simulink model "Frenet_Coordinate_State"  (R2021b)
settings: Solver=VariableStepAuto  StartTime=0.0  StopTime=10.0  RelTol=1e-3
libraries: PreScanUsefulBlocks x1, simulink x1
settings Model: Creator=admin  LastModifiedBy=admin

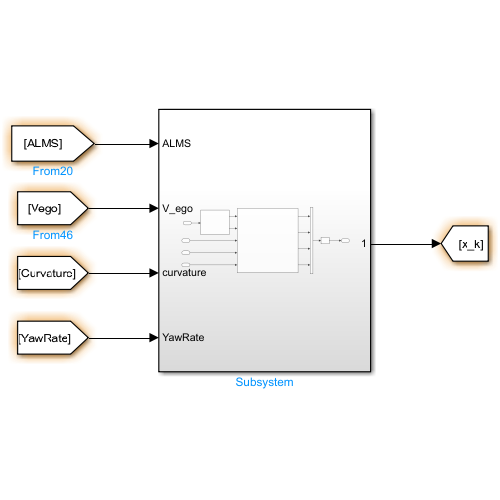
[thumbnail: Simulink's stored preview of the top-level diagram]
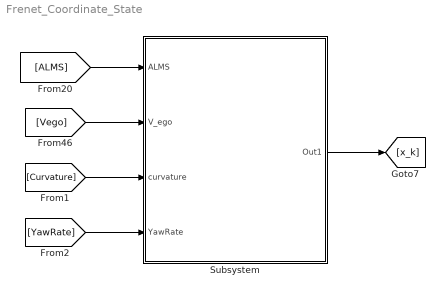
== system Frenet_Coordinate_State ==
  Subsystem : Subsystem
  wires:
  [ALMS] -> Subsystem/1(ALMS)
  [Vego] -> Subsystem/2(V_ego)
  [Curvature] -> Subsystem/3(curvature)
  [YawRate] -> Subsystem/4(YawRate)
  Subsystem/1(Out1) -> [x_k]

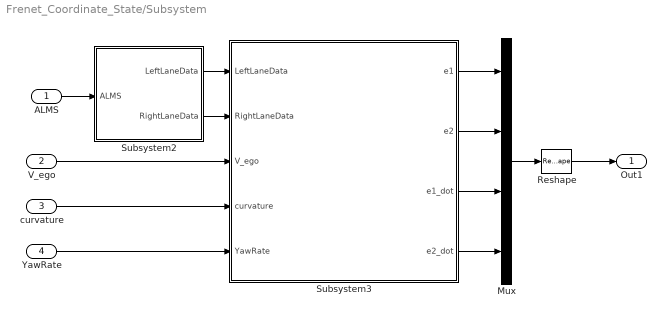
== system Frenet_Coordinate_State/Subsystem ==
  ALMS : Inport
  V_ego : Inport  Port=2
  curvature : Inport  Port=3
  YawRate : Inport  Port=4
  Mux : Mux
  Reshape : Reshape  OutputDimensionality=Customize  OutputDimensions=[4,1]
  Subsystem2 : Subsystem
  Subsystem3 : Subsystem
  Out1 : Outport
  wires:
  Subsystem3/1(e1) -> Mux/1
  Reshape/1 -> Out1/1
  Subsystem3/3(e1_dot) -> Mux/3
  Subsystem3/4(e2_dot) -> Mux/4
  Subsystem2/2(RightLaneData) -> Subsystem3/2(RightLaneData)
  Subsystem3/2(e2) -> Mux/2
  Mux/1 -> Reshape/1
  Subsystem2/1(LeftLaneData) -> Subsystem3/1(LeftLaneData)
  YawRate/1 -> Subsystem3/5(YawRate)
  V_ego/1 -> Subsystem3/3(V_ego)
  ALMS/1 -> Subsystem2/1(ALMS)
  curvature/1 -> Subsystem3/4(curvature)

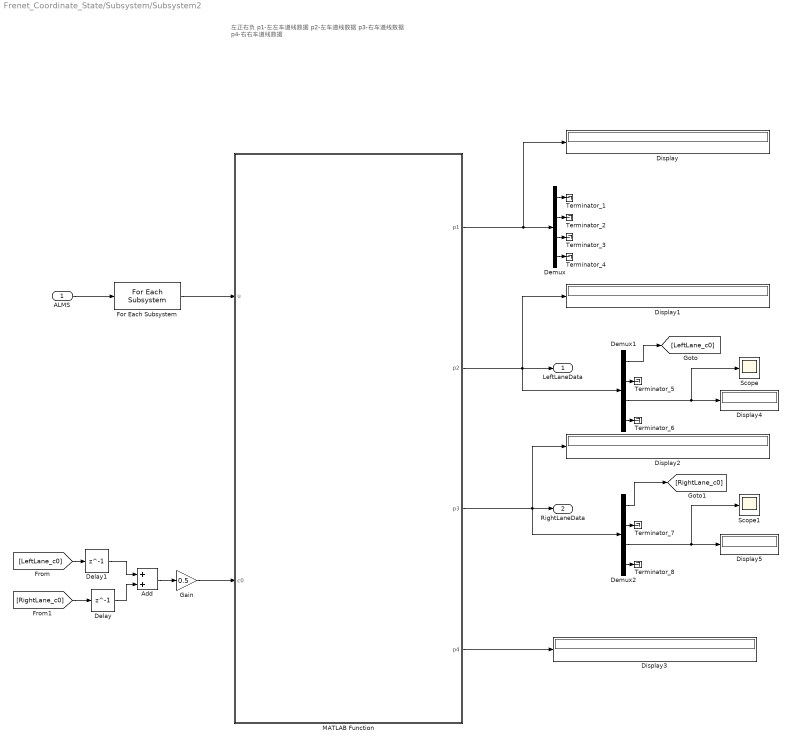
== system Frenet_Coordinate_State/Subsystem/Subsystem2 ==
  note: 左正右负
      | p1-左左车道线数据
      | p2-左车道线数据
      | p3-右车道线数据
      | p4-右右车道线数据
  ALMS : Inport  OutDataTypeStr=Bus: PRESCAN_ALMS_MESSAGE
  Add : Sum
  Delay : Delay  DelayLength=1
  Delay1 : Delay  DelayLength=1
  Demux : Demux
  Demux1 : Demux
  Demux2 : Demux
  Display{,1..5} (6 alike) : Display
  For Each Subsystem : PreScanUsefulBlocks/ALMS XY Polynomial Plot/For Each Subsystem  SystemSampleTime=-1  VariantActivationTime=update diagram  Latency=0  AutoFrameSizeCalculation=off
  Gain : Gain  Gain=0.5
  MATLAB Function : MATLAB Function  TreatAsAtomicUnit=on
  Scope : Scope
  Scope1 : Scope
  Terminator_{1..8} (8 alike) : Terminator
  LeftLaneData : Outport  VectorParamsAs1DForOutWhenUnconnected=off
  RightLaneData : Outport  Port=2  VectorParamsAs1DForOutWhenUnconnected=off
  wires:
  For Each Subsystem/1 -> MATLAB Function/1(u)
  ALMS/1 -> For Each Subsystem/1
  Gain/1 -> MATLAB Function/2(c0)
  Demux1/3 -> Scope/1, Display4/1
  Demux2/3 -> Scope1/1, Display5/1
  Demux1/1 -> [LeftLane_c0]
  Demux2/1 -> [RightLane_c0]
  [LeftLane_c0] -> Delay1/1
  [RightLane_c0] -> Delay/1
  Add/1 -> Gain/1
  Delay1/1 -> Add/1
  Delay/1 -> Add/2
  MATLAB Function/2(p2) -> Demux1/1, LeftLaneData/1, Display1/1
  MATLAB Function/1(p1) -> Display/1, Demux/1
  MATLAB Function/3(p3) -> Demux2/1, RightLaneData/1, Display2/1
  MATLAB Function/4(p4) -> Display3/1
  Demux/1 -> Terminator_1/1
  Demux/2 -> Terminator_2/1
  Demux/3 -> Terminator_3/1
  Demux/4 -> Terminator_4/1
  Demux1/2 -> Terminator_5/1
  Demux1/4 -> Terminator_6/1
  Demux2/2 -> Terminator_7/1
  Demux2/4 -> Terminator_8/1

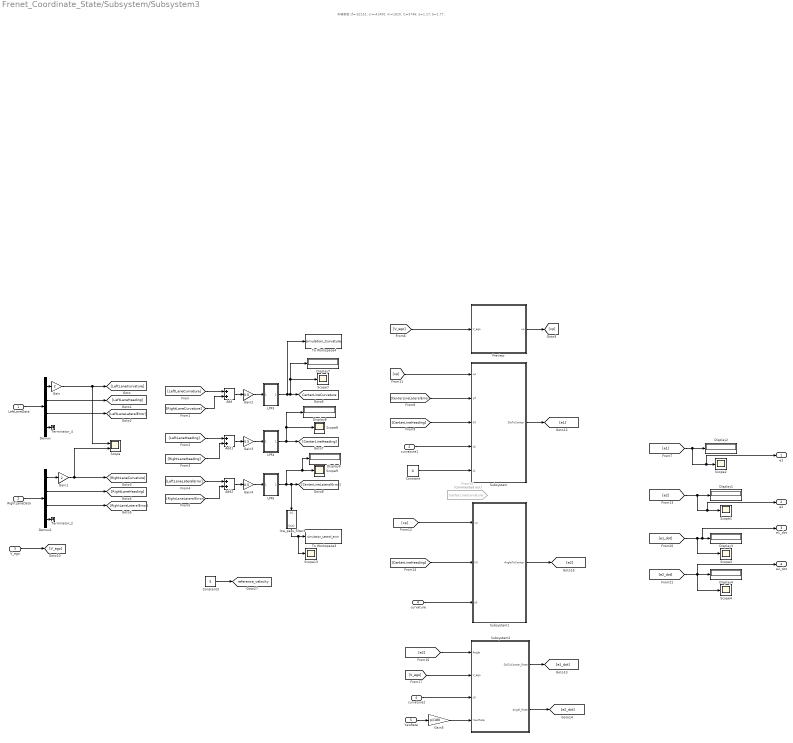
== system Frenet_Coordinate_State/Subsystem/Subsystem3 ==
  note: 车辆参数
      | cf=-52151;
      | cr=-41400;
      | m=1820;
      | Iz=3746;
      | a=1.17;
      | b=1.77;
  LeftLaneData : Inport
  RightLaneData : Inport  Port=2
  V_ego : Inport  Port=3
  curvature : Inport  Port=4
  YawRate : Inport  Port=5
  Add : Sum
  Add1 : Sum
  Add2 : Sum
  Constant : Constant  Value=0
  Constant3 : Constant  Value=5
  Demux : Demux
  Demux1 : Demux
  Display{1..4,7..9} (7 alike) : Display
  From10 : From  Commented=on  GotoTag=CenterLineCurvature  TagVisibility=global
  Gain : Gain  Gain=2
  Gain1 : Gain  Gain=2
  Gain2 : Gain  Gain=0.5
  Gain3 : Gain  Gain=0.5
  Gain4 : Gain  Gain=0.5
  Gain5 : Gain  Gain=pi/180
  LPF3 : Subsystem
  LPF4 : Subsystem
  LPF5 : Subsystem
  Preview : Subsystem
  Scope : Scope  NumInputPorts=2
  Scope{1..4,7..9,13} (8 alike) : Scope
  Subsystem : Subsystem
  Subsystem1 : Subsystem
  Subsystem2 : Subsystem
  Terminator_2 : Terminator
  Terminator_4 : Terminator
  To Workspace3 : ToWorkspace  VariableName=simulation_Lateral_error  SampleTime=-1
      settings: Save2DSignal=2-D array (concatenate along first dimension)
  To Workspace4 : ToWorkspace  VariableName=simulation_Curvature  SampleTime=-1
      settings: Save2DSignal=2-D array (concatenate along first dimension)
  curvature1 : InportShadow  Port=4
  curvature2 : InportShadow  Port=4
  low_pass_filter3 : Subsystem
  e1 : Outport
  e2 : Outport  Port=2
  e1_dot : Outport  Port=3
  e2_dot : Outport  Port=4
  tag scope: CenterLineCurvature=global, reference_velocity=global
  wires:
  LeftLaneData/1 -> Demux/1
  RightLaneData/1 -> Demux1/1
  Demux/1 -> Gain/1
  Demux1/1 -> Gain1/1
  [LeftLaneCurvature] -> Add/1
  [RightLaneCurvature] -> Add/2
  Add/1 -> Gain2/1
  Gain2/1 -> LPF3/1(In1)
  Add1/1 -> Gain3/1
  [LeftLaneHeading] -> Add1/1
  [RightLaneHeading] -> Add1/2
  [LeftLaneLateralError] -> Add2/1
  [RightLaneLateralError] -> Add2/2
  Add2/1 -> Gain4/1
  V_ego/1 -> [V_ego]
  [V_ego] -> Preview/1(V_ego)
  [CenterLineLateralError] -> Subsystem/2(y0)
  [CenterLineHeading] -> Subsystem/3(k0)
  Constant/1 -> Subsystem/5(c1)
  [xp] -> Subsystem/1(xp)
  [xp] -> Subsystem1/1(xp)
  [CenterLineHeading] -> Subsystem1/2(k0)
  [e2] -> Subsystem2/1(Angle)
  [V_ego] -> Subsystem2/2("V_ego ")
  YawRate/1 -> Gain5/1
  Subsystem/1(DisToCenter) -> [e1]
  Subsystem1/1(AngleToCenter) -> [e2]
  Subsystem2/1(DisToCenter_Rate) -> [e1_dot]
  Subsystem2/2(Angel_Rate) -> [e2_dot]
  Gain3/1 -> LPF4/1(In1)
  Gain4/1 -> LPF5/1(In1)
  Gain/1 -> Scope/1, [LeftLaneCurvature]
  Demux/2 -> [LeftLaneHeading]
  Demux/3 -> [LeftLaneLateralError]
  Gain1/1 -> Scope/2, [RightLaneCurvature]
  Demux1/2 -> [RightLaneHeading]
  Demux1/3 -> [RightLaneLateralError]
  LPF3/1(Out1) -> To Workspace4/1, Display7/1, Scope7/1, [CenterLineCurvature]
  LPF4/1(Out1) -> [CenterLineHeading], Display8/1, Scope8/1
  LPF5/1(Out1) -> [CenterLineLateralError], low_pass_filter3/1(In1), Display9/1, Scope9/1
  Demux/4 -> Terminator_4/1
  Demux1/4 -> Terminator_2/1
  Preview/1(xp) -> [xp]
  Gain5/1 -> Subsystem2/4(YawRate)
  low_pass_filter3/1(Out1) -> Scope13/1, To Workspace3/1
  Constant3/1 -> [reference_velocity]
  [e1] -> e1/1, Scope2/1, Display2/1
  [e2] -> Display1/1, e2/1, Scope1/1
  [e1_dot] -> Scope3/1, e1_dot/1, Display3/1
  [e2_dot] -> e2_dot/1, Display4/1, Scope4/1
  curvature1/1 -> Subsystem/4(c0)
  curvature/1 -> Subsystem1/3(c0)
  curvature2/1 -> Subsystem2/3(c0)

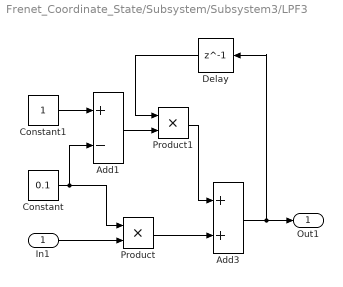
== system Frenet_Coordinate_State/Subsystem/Subsystem3/LPF3 ==
  In1 : Inport
  Add1 : Sum  Inputs=+-
  Add3 : Sum
  Constant : Constant  Value=0.1
  Constant1 : Constant
  Delay : Delay  DelayLength=1
  Product : Product
  Product1 : Product
  Out1 : Outport  VectorParamsAs1DForOutWhenUnconnected=off
  wires:
  In1/1 -> Product/2
  Add3/1 -> Delay/1, Out1/1
  Product/1 -> Add3/2
  Constant/1 -> Add1/2, Product/1
  Constant1/1 -> Add1/1
  Add1/1 -> Product1/2
  Delay/1 -> Product1/1
  Product1/1 -> Add3/1

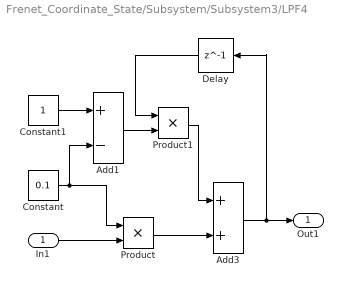
== system Frenet_Coordinate_State/Subsystem/Subsystem3/LPF4 ==
  In1 : Inport
  Add1 : Sum  Inputs=+-
  Add3 : Sum
  Constant : Constant  Value=0.1
  Constant1 : Constant
  Delay : Delay  DelayLength=1
  Product : Product
  Product1 : Product
  Out1 : Outport  VectorParamsAs1DForOutWhenUnconnected=off
  wires:
  Product1/1 -> Add3/1
  Delay/1 -> Product1/1
  Add1/1 -> Product1/2
  Constant1/1 -> Add1/1
  Constant/1 -> Product/1, Add1/2
  Product/1 -> Add3/2
  Add3/1 -> Out1/1, Delay/1
  In1/1 -> Product/2

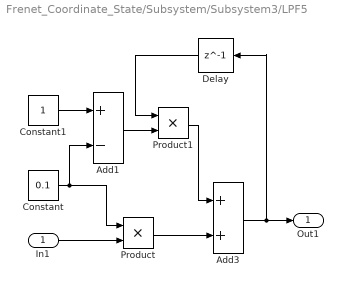
== system Frenet_Coordinate_State/Subsystem/Subsystem3/LPF5 ==
  In1 : Inport
  Add1 : Sum  Inputs=+-
  Add3 : Sum
  Constant : Constant  Value=0.1
  Constant1 : Constant
  Delay : Delay  DelayLength=1
  Product : Product
  Product1 : Product
  Out1 : Outport  VectorParamsAs1DForOutWhenUnconnected=off
  wires:
  In1/1 -> Product/2
  Add3/1 -> Delay/1, Out1/1
  Product/1 -> Add3/2
  Constant/1 -> Add1/2, Product/1
  Constant1/1 -> Add1/1
  Add1/1 -> Product1/2
  Delay/1 -> Product1/1
  Product1/1 -> Add3/1

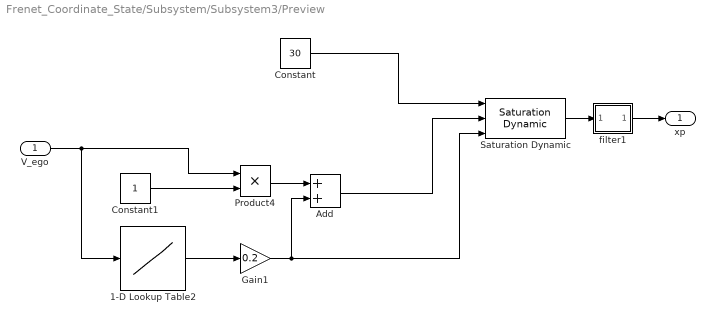
== system Frenet_Coordinate_State/Subsystem/Subsystem3/Preview ==
  V_ego : Inport
  1-D Lookup Table2 : Lookup_n-D  NumberOfTableDimensions=1  BreakpointsForDimension1=[0,3,5,10,15,20,30,40,50]  Table=[6,6,7,8.5,10.5,12,14,15,15]  InternalRulePriority=Speed  RndMeth=Simplest  InputSameDT=on
  Add : Sum
  Constant : Constant  Value=30
  Constant1 : Constant
  Gain1 : Gain  Gain=0.2
  Product4 : Product
  Saturation Dynamic : simulink/Discontinuities/Saturation Dynamic  OutMin=[]  OutMax=[]  OutDataTypeStr=Inherit: Same as second input  OutDataType=fixdt(1, 16)  OutScaling=2^-10  DoSatur=off
  filter1 : Subsystem
  xp : Outport  VectorParamsAs1DForOutWhenUnconnected=off
  wires:
  Constant/1 -> Saturation Dynamic/1
  Saturation Dynamic/1 -> filter1/1(In1)
  V_ego/1 -> 1-D Lookup Table2/1, Product4/1
  Product4/1 -> Add/1
  1-D Lookup Table2/1 -> Gain1/1
  Gain1/1 -> Add/2, Saturation Dynamic/3
  Constant1/1 -> Product4/2
  filter1/1(Out1) -> xp/1
  Add/1 -> Saturation Dynamic/2

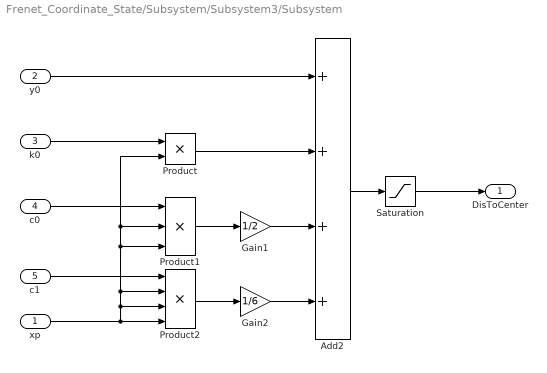
== system Frenet_Coordinate_State/Subsystem/Subsystem3/Subsystem ==
  xp : Inport
  y0 : Inport  Port=2
  k0 : Inport  Port=3
  c0 : Inport  Port=4
  c1 : Inport  Port=5
  Add2 : Sum  Inputs=++++
  Gain1 : Gain  Gain=1/2
  Gain2 : Gain  Gain=1/6
  Product : Product
  Product1 : Product  Inputs=3
  Product2 : Product  Inputs=4
  Saturation : Saturate  UpperLimit=3.5  LowerLimit=-3.5
  DisToCenter : Outport  VectorParamsAs1DForOutWhenUnconnected=off
  wires:
  Product1/1 -> Gain1/1
  Product2/1 -> Gain2/1
  Product/1 -> Add2/2
  c1/1 -> Product2/1
  Gain1/1 -> Add2/3
  Gain2/1 -> Add2/4
  c0/1 -> Product1/1
  Add2/1 -> Saturation/1
  xp/1 -> Product2/4, Product2/3, Product2/2, Product1/3, Product1/2, Product/2
  y0/1 -> Add2/1
  k0/1 -> Product/1
  Saturation/1 -> DisToCenter/1

== system Frenet_Coordinate_State/Subsystem/Subsystem3/Subsystem1 ==
  xp : Inport
  k0 : Inport  Port=2
  c0 : Inport  Port=3
  Add2 : Sum
  Product1 : Product
  Trigonometric Function : Trigonometry  Operator=atan
  AngleToCenter : Outport  VectorParamsAs1DForOutWhenUnconnected=off
  wires:
  Trigonometric Function/1 -> AngleToCenter/1
  c0/1 -> Product1/1
  Add2/1 -> Trigonometric Function/1
  Product1/1 -> Add2/2
  k0/1 -> Add2/1
  xp/1 -> Product1/2

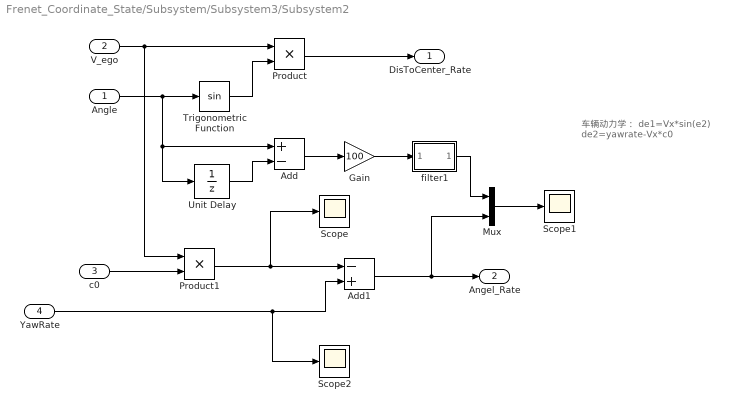
== system Frenet_Coordinate_State/Subsystem/Subsystem3/Subsystem2 ==
  note: 车辆动力学：
      | de1=Vx*sin(e2)
      | de2=yawrate-Vx*c0
  Angle : Inport
  "V_ego " : Inport  Port=2
  c0 : Inport  Port=3
  YawRate : Inport  Port=4
  Add : Sum  Inputs=+-
  Add1 : Sum  Inputs=-+
  Gain : Gain  Gain=100
  Mux : Mux  Inputs=2
  Product : Product
  Product1 : Product
  Scope : Scope
  Scope1 : Scope
  Scope2 : Scope
  Trigonometric Function : Trigonometry
  Unit Delay : UnitDelay  SampleTime=-1  HasFrameUpgradeWarning=on
  filter1 : Subsystem
  DisToCenter_Rate : Outport  VectorParamsAs1DForOutWhenUnconnected=off
  Angel_Rate : Outport  Port=2  VectorParamsAs1DForOutWhenUnconnected=off
  wires:
  "V_ego "/1 -> Product1/1, Product/1
  Angle/1 -> Unit Delay/1, Add/1, Trigonometric Function/1
  Product/1 -> DisToCenter_Rate/1
  Trigonometric Function/1 -> Product/2
  Unit Delay/1 -> Add/2
  Add/1 -> Gain/1
  Gain/1 -> filter1/1(In1)
  Mux/1 -> Scope1/1
  c0/1 -> Product1/2
  Product1/1 -> Scope/1, Add1/1
  Add1/1 -> Angel_Rate/1, Mux/2
  filter1/1(Out1) -> Mux/1
  YawRate/1 -> Scope2/1, Add1/2

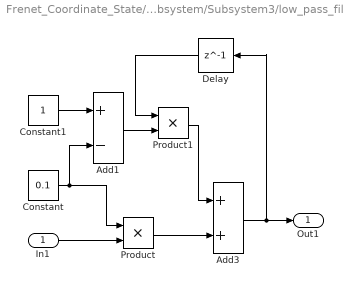
== system Frenet_Coordinate_State/Subsystem/Subsystem3/low_pass_filter3 ==
  In1 : Inport
  Add1 : Sum  Inputs=+-
  Add3 : Sum
  Constant : Constant  Value=0.1
  Constant1 : Constant
  Delay : Delay  DelayLength=1
  Product : Product
  Product1 : Product
  Out1 : Outport  VectorParamsAs1DForOutWhenUnconnected=off
  wires:
  Product1/1 -> Add3/1
  Delay/1 -> Product1/1
  Add1/1 -> Product1/2
  Constant1/1 -> Add1/1
  Constant/1 -> Product/1, Add1/2
  Product/1 -> Add3/2
  Add3/1 -> Out1/1, Delay/1
  In1/1 -> Product/2

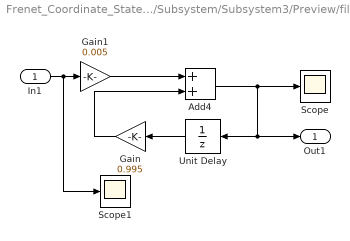
== system Frenet_Coordinate_State/Subsystem/Subsystem3/Preview/filter1 ==
  In1 : Inport
  Add4 : Sum
  Gain : Gain  Gain=0.995
  Gain1 : Gain  Gain=0.005
  Scope : Scope
  Scope1 : Scope
  Unit Delay : UnitDelay  InitialCondition=30  SampleTime=-1  HasFrameUpgradeWarning=on
  Out1 : Outport  VectorParamsAs1DForOutWhenUnconnected=off
  wires:
  Gain1/1 -> Add4/1
  Gain/1 -> Add4/2
  Unit Delay/1 -> Gain/1
  Add4/1 -> Unit Delay/1, Out1/1, Scope/1
  In1/1 -> Scope1/1, Gain1/1

== system Frenet_Coordinate_State/Subsystem/Subsystem3/Subsystem2/filter1 ==
  In1 : Inport
  Add4 : Sum
  Gain : Gain  Gain=0.9
  Gain1 : Gain  Gain=0.1
  Scope : Scope
  Unit Delay : UnitDelay  SampleTime=-1  HasFrameUpgradeWarning=on
  Out1 : Outport  VectorParamsAs1DForOutWhenUnconnected=off
  wires:
  Gain1/1 -> Add4/1
  Gain/1 -> Add4/2
  In1/1 -> Gain1/1
  Unit Delay/1 -> Gain/1
  Add4/1 -> Unit Delay/1, Out1/1, Scope/1

== matlab function Frenet_Coordinate_State/Subsystem/Subsystem2/MATLAB Function ==
  settings: updateMethod=DISCRETE  sampleTime=1/20
  data: u input; c0 input; p1 output; p2 output; p3 output; p4 output
function [p1,p2,p3,p4]=fcn(u,c0)
p1=zeros(1,4);p2=zeros(1,4)';p3=zeros(1,4)';p4=zeros(1,4);
coder.extrinsic('polyval','plot','axis','hold','drawnow','fcn_setCurrentFigureNoFocus','set','clf','figure','ishandle','xlabel','ylabel');

index = 0;
lanedata=zeros(600,3);  %%车道线数据
for i = 1 : length(u)/12
    if u(index+1) == 1
        in = struct(...
            'valid',u(index+1), ...
            'XN0',u(index+2), ...
            'XN1',u(index+3), ...
            'XN2',u(index+4), ...
            'XN3',u(index+5), ...
            'YN0',u(index+6), ...
            'YN1',u(index+7), ...
            'YN2',u(index+8), ...
            'YN3',u(index+9), ...
            'Length',u(index+10), ...
            'GroupID',u(index+11), ...
            'LineLabel',u(index+12) ...
        );
        
        % Construct polynomial definitions 
        Px = [in.XN3, in.XN2, in.XN1, in.XN0];
        Py = [in.YN3, in.YN2, in.YN1, in.YN0];
        
        % Extract polynomial interval
        L1 = 0;
        L2 = in.Length;
        n=30;
        L = linspace(L1,L2,n);
        x=zeros(1,n);y=zeros(1,n);
        x = polyval(Px,L);
        y = polyval(Py,L);   
 %%%对ALMS输出的20段线进行筛选       
        lanedata(i*30-29:30*i,1)= x;
        lanedata(i*30-29:30*i,2)= y;  
        if abs(mean(y-0.5*c0*x.^2+5.25))<=1          %%右右车道线   ，mean求解数组平均值
            lanedata(i*30-29:30*i,3)=4;
        elseif abs(mean(y-0.5*c0*x.^2+1.75))<=1   %%右车道线
            lanedata(i*30-29:30*i,3)=3;
        elseif abs(mean(y-0.5*c0*x.^2-1.75))<=1    %%左车道线
            lanedata(i*30-29:30*i,3)=2;
        elseif abs(mean(y-0.5*c0*x.^2-5.25))<=1    %%左左车道线
            lanedata(i*30-29:30*i,3)=1;
        end       
    end
    index = index + 12;
end

%%%ALMS输出车道线的拟合参数
pfit=zeros(4,4);
for i=1:4
laneindex=find(lanedata(:,3)==i);
if ~isempty(laneindex)
    X=lanedata(laneindex,1);Y=lanedata(laneindex,2);
    pfit(i,:)=[polyfit(X,Y,2),i];
end
end
p1=pfit(1,:);p2=pfit(2,:)';p3=pfit(3,:)';p4=pfit(4,:);
